simulink model "Simulink_Practica_6"  (R2022b)
settings: Solver=VariableStepAuto  StartTime=0.0  StopTime=0.01  RelTol=1e-3
values from neighbouring files (symbols this model uses):
  C = 10e-6    (= 1e-05)    [CD.m]    (also in Parametros_P6.m)
  L = 2e-3    (= 0.002)    [CD.m]    (also in Parametros_P6.m)
  R = 10    [CD.m]    (also in Parametros_P6.m)
  Vin = 32    [CD.m]    (also in Parametros_P6.m)
settings Model: Creator=escor  LastModifiedBy=escor

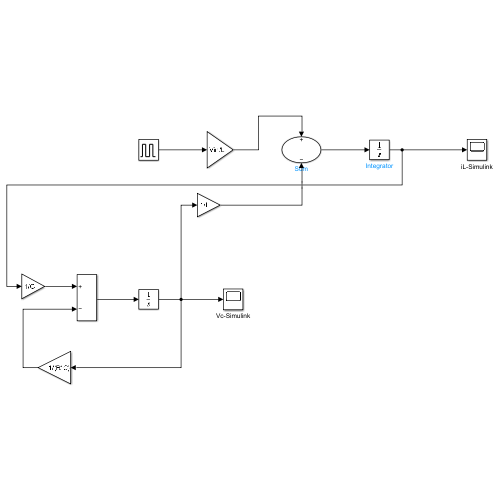
[thumbnail: Simulink's stored preview of the top-level diagram]
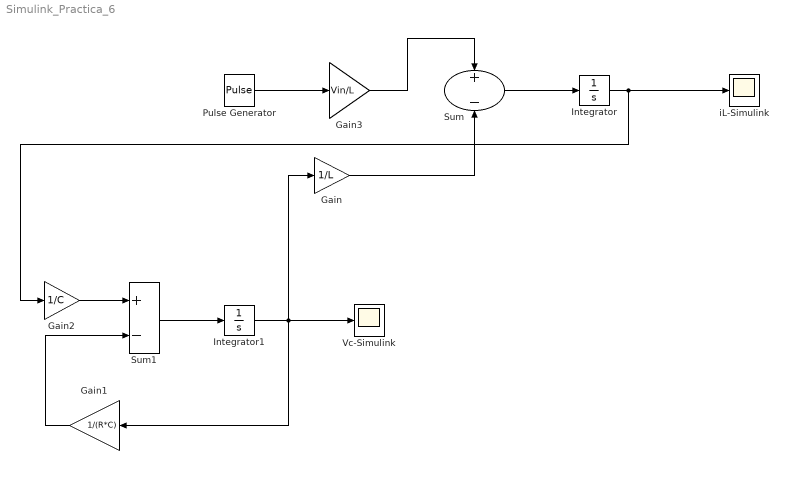
== system Simulink_Practica_6 ==
  Gain : Gain  Gain=1/L
  Gain1 : Gain  Gain=1/(R*C)
  Gain2 : Gain  Gain=1/C
  Gain3 : Gain  Gain=Vin/L
  Integrator : Integrator
  Integrator1 : Integrator
  Pulse Generator : DiscretePulseGenerator  PulseType=Time based  Amplitude=0.955  Period=1e-5  PulseWidth=40
  Sum : Sum  Inputs=+-
  Sum1 : Sum  Inputs=+-
  Vc-Simulink : Scope
  iL-Simulink : Scope
  wires:
  Sum/1 -> Integrator/1
  Gain3/1 -> Sum/1
  Sum1/1 -> Integrator1/1
  Pulse Generator/1 -> Gain3/1
  Integrator1/1 -> Gain/1, Vc-Simulink/1, Gain1/1
  Gain2/1 -> Sum1/1
  Gain1/1 -> Sum1/2
  Gain/1 -> Sum/2
  Integrator/1 -> Gain2/1, iL-Simulink/1
